simulink model "multi_ISO"  (R2018b)
settings: Solver=VariableStepAuto  StartTime=0.0  StopTime=10.0  RelTol=1e-3
settings Model: Creator=kekos  LastModifiedBy=kekos

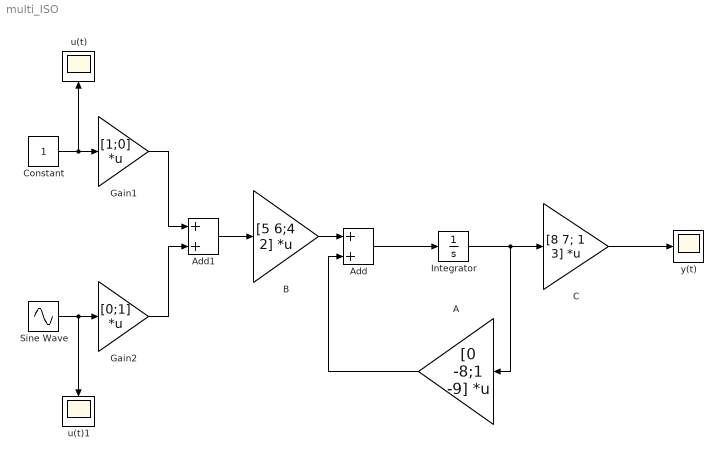
== system multi_ISO ==
  " u(t)" : Scope
  " u(t)1" : Scope
  A : Gain  Gain=[0 -8;1 -9]  Multiplication=Matrix(K*u)
  Add : Sum
  Add1 : Sum
  B : Gain  Gain=[5 6;4 2]  Multiplication=Matrix(K*u)
  "C " : Gain  Gain=[8 7; 1 3]  Multiplication=Matrix(K*u)
  Constant : Constant
  Gain1 : Gain  Gain=[1;0]  Multiplication=Matrix(K*u)
  Gain2 : Gain  Gain=[0;1]  Multiplication=Matrix(K*u)
  Integrator : Integrator  InitialCondition=[0.6;0.2]
  Sine Wave : Sin  Amplitude=2  SampleTime=0
  y(t) : Scope
  wires:
  B/1 -> Add/1
  "C "/1 -> y(t)/1
  Add/1 -> Integrator/1
  A/1 -> Add/2
  Integrator/1 -> A/1, "C "/1
  Add1/1 -> B/1
  Gain2/1 -> Add1/2
  Gain1/1 -> Add1/1
  Constant/1 -> " u(t)"/1, Gain1/1
  Sine Wave/1 -> " u(t)1"/1, Gain2/1
